simulink model "Isolated_Full_Bridge_DC_DC_Converter_2"  (R2021a)
settings: Solver=VariableStepAuto  StartTime=0.0  StopTime=0.01  RelTol=1e-3
libraries: spsCurrentMeasurementLib x5, spsMosfetLib x4, spsVoltageMeasurementLib x4, spsSeriesRLCBranchLib x3, spsDiodeLib x2, spsLinearTransformerLib x1, dspstat3 x1, spsDCVoltageSourceLib x1, spspowerguiLib x1
settings Model: Creator=EREN-PC  LastModifiedBy=EREN-PC

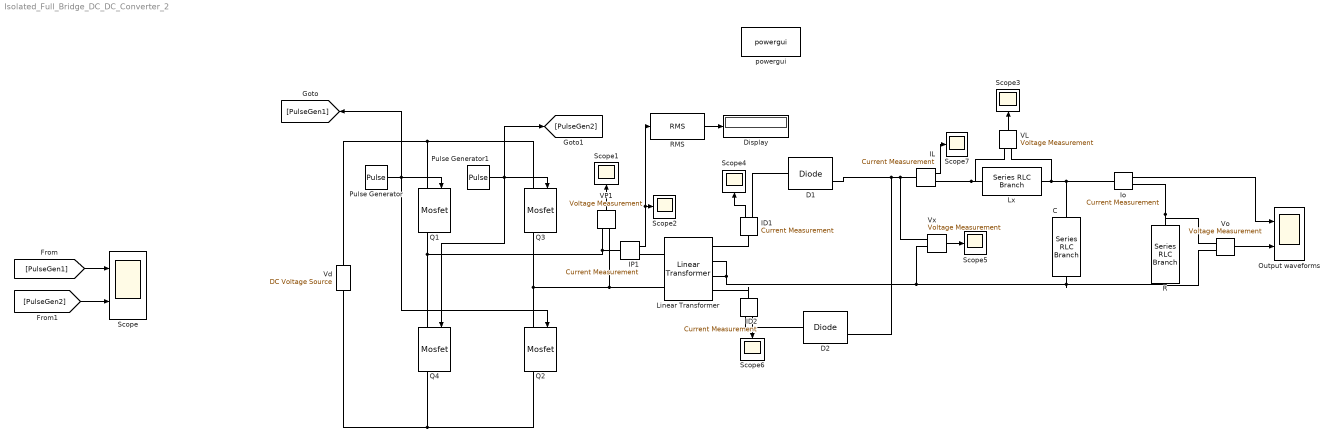
== system Isolated_Full_Bridge_DC_DC_Converter_2 ==
  C : spsSeriesRLCBranchLib/Series RLC Branch  LConnTagsString=__new0  RConnTagsString=__new0  BranchType=C  Resistance=1  Inductance=240e-6  SetiL0=off  InitialCurrent=0  Capacitance=260e-6  Setx0=off  InitialVoltage=0  Measurements=None
  D1 : spsDiodeLib/Diode  Ron=0.001  Lon=0  Vf=0  IC=0  UseSnubber=0  Rs=500  Cs=250e-9  Measurements=on
  D2 : spsDiodeLib/Diode  Ron=0.001  Lon=0  Vf=0  IC=0  UseSnubber=0  Rs=500  Cs=250e-9  Measurements=on
  Display : Display
  ID1 : spsCurrentMeasurementLib/Current Measurement  PhasorSimulation=off  OutputType=Complex  PSBequivalent=0
  ID2 : spsCurrentMeasurementLib/Current Measurement  PhasorSimulation=off  OutputType=Complex  PSBequivalent=0
  IL : spsCurrentMeasurementLib/Current Measurement  PhasorSimulation=off  OutputType=Complex  PSBequivalent=0
  IP1 : spsCurrentMeasurementLib/Current Measurement  PhasorSimulation=off  OutputType=Complex  PSBequivalent=0
  Io : spsCurrentMeasurementLib/Current Measurement  PhasorSimulation=off  OutputType=Complex  PSBequivalent=0
  Linear Transformer : spsLinearTransformerLib/Linear Transformer  UNITS=SI  NominalPower=[ 96 100e3 ]  winding1=[12 0 0]  winding2=[60 0 0]  ThreeWindings=on  winding3=[60 0 0]  RmLm=[10 50.4e-6]  Measurements=None  DataType=on
  Lx : spsSeriesRLCBranchLib/Series RLC Branch  LConnTagsString=__new0  RConnTagsString=__new0  BranchType=L  Resistance=1  Inductance=240e-6  SetiL0=off  InitialCurrent=0  Capacitance=1e-6  Setx0=off  InitialVoltage=0  Measurements=None
  Output waveforms : Scope  NumInputPorts=2
  Pulse Generator : DiscretePulseGenerator  PulseType=Time based  Period=1/100000  PulseWidth=50
  Pulse Generator1 : DiscretePulseGenerator  PulseType=Time based  Period=1/100000  PulseWidth=50  PhaseDelay=1/200000
  Q{1..4} (4 alike) : spsMosfetLib/Mosfet  Ron=0.1  Lon=0  Rd=0.01  Vfd=0  IC=0  Rs=1e5  Cs=inf  Measurements=on
  R : spsSeriesRLCBranchLib/Series RLC Branch  LConnTagsString=__new0  RConnTagsString=__new0  BranchType=R  Resistance=24  Inductance=1e-3  SetiL0=off  InitialCurrent=0  Capacitance=1e-6  Setx0=off  InitialVoltage=0  Measurements=None
  RMS : dspstat3/RMS  run=off  directionMode=Each column  dimension=1  InputProcessing=Columns as channels (frame based)  reset_popup=None
  Scope : Scope  NumInputPorts=2
  Scope{1..7} (7 alike) : Scope
  VL : spsVoltageMeasurementLib/Voltage Measurement  PhasorSimulation=off  OutputType=Complex  PSBequivalent=0
  VP1 : spsVoltageMeasurementLib/Voltage Measurement  PhasorSimulation=off  OutputType=Complex  PSBequivalent=0
  Vd : spsDCVoltageSourceLib/DC Voltage Source  Amplitude=12  Measurements=None
  Vo : spsVoltageMeasurementLib/Voltage Measurement  PhasorSimulation=off  OutputType=Complex  PSBequivalent=0
  Vx : spsVoltageMeasurementLib/Voltage Measurement  PhasorSimulation=off  OutputType=Complex  PSBequivalent=0
  powergui : spspowerguiLib/powergui  Priority=1  SimulationMode=Continuous  SampleTime=50e-6  frequency=60  Iterations=50  frequencyindice=0  Pbase=100e6  ErrMax=1e-4  UnitsV=kV  UnitsW=MW  buscounter=0  FunctionMessages=off  echomessages=off  EnableUseOfTLC=off  CurrentSourceSwitches=off  DisableSnubberDevices=off  DisableRonSwitches=off  DisableVfSwitches=off  DisplayEquations=off  AutomaticDiscreteSolvers=off  SolverType=Tustin/Backward Euler (TBE)  Interpol=off  ExternalGateDelay=off  methode=off  Ts=100  x0status=blocks  SPID=on  SwTol=0  HookPort=off  NonlinearTolerance=1e-4  nMaxIteration=100  ContinueOnMaxIteration=off  RestoreLinks=warning  ResistiveCurrentMeasurement=off  Frange=[0:2:500]  Ylog=off  Xlog=on  ShowGrid=off  save=off  variable=ZData  structure=0  ZoomFFT=off  StartTime=0.0  cycles=1  DisplayStyle=1  fundamental=60  FreqAxis=off  MaxFrequency=1000  frequencyindicesteady=1  RmsSteady=1  display=off
  wires:
  Pulse Generator/1 -> [PulseGen1], Q2/1, Q1/1
  Pulse Generator1/1 -> [PulseGen2], Q4/1, Q3/1
  [PulseGen1] -> Scope/1
  [PulseGen2] -> Scope/2
  Io/1 -> Output waveforms/1
  Vo/1 -> Output waveforms/2
  VP1/1 -> Scope1/1
  VL/1 -> Scope3/1
  Vx/1 -> Scope5/1
  IP1/1 -> Scope2/1, RMS/1
  RMS/1 -> Display/1
  ID1/1 -> Scope4/1
  ID2/1 -> Scope6/1
  IL/1 -> Scope7/1
  connections:
  Vd/RConn1 -- Q1/LConn1 -- Q3/LConn1
  Q4/RConn1 -- Vd/LConn1 -- Q2/RConn1
  Q3/RConn1 -- VP1/LConn2 -- Linear Transformer/LConn2 -- Q2/LConn1
  Q4/LConn1 -- IP1/LConn1 -- VP1/LConn1 -- Q1/RConn1
  Io/RConn1 -- Vo/LConn1 -- R/LConn1
  Vx/LConn1 -- IL/LConn1 -- D2/RConn1 -- D1/RConn1
  C/RConn1 -- Linear Transformer/RConn3 -- Linear Transformer/RConn2 -- Vx/LConn2 -- R/RConn1 -- Vo/LConn2
  C/LConn1 -- VL/LConn2 -- Lx/RConn1 -- Io/LConn1
  IP1/RConn1 -- Linear Transformer/LConn1
  ID1/LConn1 -- Linear Transformer/RConn1
  ID1/RConn1 -- D1/LConn1
  ID2/RConn1 -- D2/LConn1
  ID2/LConn1 -- Linear Transformer/RConn4
  VL/LConn1 -- IL/RConn1 -- Lx/LConn1
